simulink model "Kaosz"  (Simulink 7.8)
settings: Solver=ode45  StartTime=0.0  StopTime=6*pi  RelTol=1e-10
libraries: vrlib x2
settings Model: Creator=valaki  LastModifiedBy=valaki

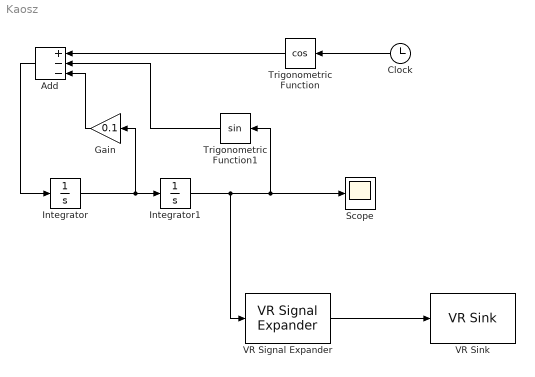
== system Kaosz ==
  Add : Sum  Inputs=+--
  Clock : Clock
  Gain : Gain  Gain=0.1
  Integrator : Integrator  InitialCondition=1.1854134
  Integrator1 : Integrator  InitialCondition=3.5145566
  Scope : Scope
  Trigonometric Function : Trigonometry  Operator=cos
  Trigonometric Function1 : Trigonometry
  VR Signal Expander : vrlib/VR Signal Expander  outwidth=4  outidx=[ 4]
  VR Sink : vrlib/VR Sink  SampleTime=0.1  ViewEnable=on  RemoteChange=off  RemoteView=off  FieldsWritten=Ball.rotation.4.1.1.double  WorldFileName=Pendulum_3D.wrl  WorldDescription=Forced Damped Pendulum  AutoView=off  VideoDimensions=[]  AllowVariableSize=off  FigureProperties="{'Position', 'Name', 'Viewpoint', 'CameraBound', 'CameraDirection', 'CameraPosition', 'CameraUpVector', 'ZoomFactor', 'Antialiasing', 'Headlight', 'Lighting', 'NavPanel', 'StatusBar', 'ToolBar', 'Textures', 'Transparency', 'Triad', 'Wireframe', 'NavZones', 'NavMode', 'NavSpeed', 'CaptureFileFormat', 'CaptureFileName', 'Record2DCompressMethod', 'Record2DCompressQuality', 'Record2D', 'Record2DFileName', 'Record2DFPS'; [5.0000000000000000e+000  9.2000000000000000e+001  5.7600000000000000e+002  3.8000000000000000e+002], 'Forced Damped Pendulum', 'Ball', 'on', [0.0000000000000000e+000  0.0000000000000000e+000 -1.0000000000000000e+000], [0.0000000000000000e+000  0.0000000000000000e+000  0.0000000000000000e+000], [0.0000000000000000e+000  1.0000000000000000e+000  0.0000000000000000e+000], [1.0000000000000000e+000], 'on', 'on', 'on', 'halfbar', 'on', 'on', 'on', 'on', 'none', 'off', 'off', 'fly', 'normal', 'tif', '%f_anim_%n.tif', 'auto', [7.5000000000000000e+001], 'off', '%f_anim_%n.avi', [1.5000000000000000e+001]}"
  wires:
  Integrator/1 -> Integrator1/1, Gain/1
  Clock/1 -> Trigonometric Function/1
  Trigonometric Function/1 -> Add/1
  Gain/1 -> Add/3
  Integrator1/1 -> Trigonometric Function1/1, Scope/1, VR Signal Expander/1
  Trigonometric Function1/1 -> Add/2
  Add/1 -> Integrator/1
  VR Signal Expander/1 -> VR Sink/1
